simulink model "Send_IMU_value_I2C"  (R2016b)
settings: Solver=FixedStepAuto  StartTime=0.0  StopTime=10.0  RelTol=1e-3
PreLoadFcn:
  | waijung.modelPreload; % Required for working with Waijung Blockset. Do not remove.
undefined symbols (not defined in the file): deg_, g, imu, Link, LQFP100, ST, STM32F407VG, STM32F4DISCOVERY
libraries: simulink x20, stm32f4_i2c_lib x8, stm32f4_io_lib x3, BC_USB x2, stm32f4_device_config_lib x1
(part 1 of 2)
CloseFcn:
  | waijung.modelClose; % Required for working with Waijung Blockset. Do not remove.
settings Model: Creator=Wall  LastModifiedBy=Wall
settings OptimizationCC: DefaultParameterBehavior=Inlined
settings DebuggingCC: ParameterTunabilityLossMsg=error
settings HardwareCC: ProdBitPerPointer=32  ProdBitPerSizeT=32  ProdBitPerPtrDiffT=32  ProdLargestAtomicFloat=None  ProdIntDivRoundTo=Undefined  ProdWordSize=32  ProdHWDeviceType=ARM Compatible->Cortex - M4  TargetEndianess=LittleEndian  TargetHWDeviceType=ARM Compatible->Cortex - M4
settings RTWCC: SystemTargetFile=stm32f4.tlc  GenerateMakefile=off  TemplateMakefile=ert_default_tmf  Description=STM32F4 Target
settings CodeAppCC: ForceParamTrailComments=on  IgnoreCustomStorageClasses=off  OperatorAnnotations=on  SimulinkDataObjDesc=on  SFDataObjDesc=on  MATLABFcnDesc=on  InsertBlockDesc=on  MATLABSourceComments=on
settings STFCustomTargetCC: TargetLangStandard=C99 (ISO)  ModelReferenceCompliant=off  CombineOutputUpdateFcns=on  ERTCustomFileBanners=on  SupportContinuousTime=off  SupportNonInlinedSFcns=off  RemoveResetFunc=on  MATLABClassNameForMDSCustomization=Simulink.SoftwareTarget.ERTCustomization  GRTInterface=off  SystemTargetFile=stm32f4.tlc
settings ERTTargetCC: TargetLangStandard=C99 (ISO)  ModelReferenceCompliant=off  ParMdlRefBuildCompliant=off  CompOptLevelCompliant=off  ConcurrentExecutionCompliant=off  ERTFirstTimeCompliant=off  ModelStepFunctionPrototypeControlCompliant=off  CPPClassGenCompliant=off  UseToolchainInfoCompliant=off  InlinedParameterPlacement=NonHierarchical  ERTSrcFileBannerTemplate=stm32f4_code_template.cgt  ERTHdrFileBannerTemplate=stm32f4_code_template.cgt  ERTDataSrcFileTemplate=stm32f4_code_template.cgt  ERTDataHdrFileTemplate=stm32f4_code_template.cgt  ERTCustomFileTemplate=stm32f4_file_process.tlc

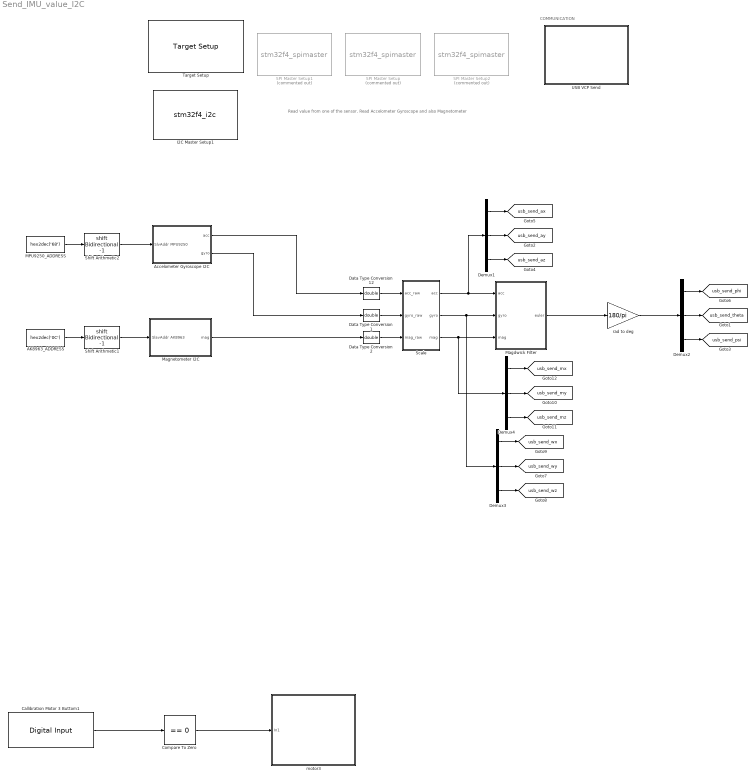
== system Send_IMU_value_I2C ==
  note: Read value from one of the sensor. Read Accelometer Gyroscope and also Magnetometer
  note: COMMUNICATION
  " AK8963_ADDRESS" : Constant  Value=hex2dec('0C')  OutDataTypeStr=uint8  SampleTime=0.002
  " MPU9250_ADDRESS" : Constant  Value=hex2dec('68')  OutDataTypeStr=uint8  SampleTime=0.002
  Accelometer Gyroscope I2C : Subsystem
  Callibration Motor 3 Buttom1 : stm32f4_io_lib/Digital Input  port=E  speed=100  porttype=Pull Up  porttypestr=UP  use_pin0=off  use_pin1=off  use_pin2=off  use_pin3=off  use_pin4=off  use_pin5=off  use_pin6=off  use_pin7=off  use_pin8=off  use_pin9=off  use_pin10=on  use_pin11=off  use_pin12=off  use_pin13=off  use_pin14=off  use_pin15=off  pinstr=GPIO_Pin_10  usedpinarray="[0  0  0  0  0  0  0  0  0  0  1  0  0  0  0  0]"  bitbandingstr="#define CallibrationMotor3Buttom1_E10 Peripheral_BB(GPIOE->IDR, 10)  /* Output pin */"  sampletime=0.002  sampletimestr=-1  blockid=CallibrationMotor3Buttom1  enablecustomportlabel=off  glabalinit=off  cinputportlabel=In1, In2  coutputportlabel=Out1, Out2
  Compare To Zero : simulink/Logic and Bit Operations/Compare To Zero  relop===  OutDataTypeStr=boolean
  Data Type Conversion1 : DataTypeConversion  OutDataTypeStr=double
  Data Type Conversion12 : DataTypeConversion  OutDataTypeStr=double
  Data Type Conversion2 : DataTypeConversion  OutDataTypeStr=double
  Demux{1..4} (4 alike) : Demux  Outputs=3
  I2C Master Setup1 : S-Function  FunctionName=stm32f4_i2c  Parameters=configuration,module,transfer,clkspeed,timeout,sdapin,sclpin,writecount,readcount,inputtypearray,outputtypearray,confstr,sampletime,sampletimestr,blockid  SFunctionDeploymentMode=off  EnableBusSupport=off  mask(stm32f4_i2c){configuration=Setup, module=1, lastmodule=1, transfer=Blocking, dutycycle=TLow/THigh = 2, clkspeed=400, timeout=25, writecount=0, readcount=0, sdapin=B9, sclpin=B6, waitwritetime=0, inputtypearray=[0], outputtypearray=[0], confstr=["B","9","B","6","1","1","6","0","I2C_DutyCycle_2","0","off"], sampletime=-1, sampletimestr=-1, blockid=I2CMasterSetup1}
      mask prompts: module "I2C Module"; lastmodule "Last module"; transfer "Transfer mode"; dutycycle "Duty cycle in fast mode"; clkspeed "Clock speed (kHz)"; timeout "Timeout (ms)"; writecount "Bytes write count"; readcount "Bytes read count"; sdapin "SDA pin"; sclpin "SCL pin"; waitwritetime "Wait write time (ms), default is 0"; inputtypearray "Input type array"; outputtypearray "Output type array"; confstr "Configuration string"; sampletime "Sample time (sec)"; sampletimestr "Compiled sample time (sec) in string"
      mask init:
      | stm32f4_i2c_callback('init');
      mask Help: web(fullfile(waijungdocroot,'stm32f4_i2c_setup.htm'), '-browser')
      mask TypeOptions configuration: Setup | Transaction
      mask Callback configuration: stm32f4_i2c_callback('configuration');
      mask TypeOptions module: 1 | 2 | 3
      mask Callback module: stm32f4_i2c_callback('module');
      mask TypeOptions transfer: Blocking | Non-blocking
      mask TypeOptions dutycycle: TLow/THigh = 16/9 | TLow/THigh = 2
      mask Callback dutycycle: stm32f4_i2c_callback('dutycycle');
      mask Callback writecount: stm32f4_i2c_callback('writecount');
      mask Callback readcount: stm32f4_i2c_callback('readcount');
      mask TypeOptions sdapin: - | B7 | B9
      mask Callback sdapin: stm32f4_i2c_callback('sdapin');
      mask TypeOptions sclpin: - | B6 | B8
      mask Callback sclpin: stm32f4_i2c_callback('sclpin');
      mask Callback confstr: stm32f4_i2c_callback('confstr');
      mask Callback sampletime: stm32f4_i2c_callback('sampletime');
      mask Callback sampletimestr: stm32f4_i2c_callback('sampletimestr');
      mask Callback blockid: stm32f4_i2c_callback('blockid');
      mask Display: text(0.5, 0.5, 'Module: I2C1\nClock: 400kHz\nSDA/SCL Pin: B9/B6','ver','middle','hor','center');
  Magdwick Filter : MATLAB Function  TreatAsAtomicUnit=on
  Magnetometer I2C : Subsystem
  SPI Master Setup : S-Function  Commented=on  FunctionName=stm32f4_spimaster  Parameters=mode,configuration,module,datacount,inputtypearray,outputtypearray,confstr,sampletime,sampletimestr,blockid  SFunctionDeploymentMode=off  EnableBusSupport=off  mask(stm32f4_spimaster){configuration=Setup, module=2, mode=Write, lastmodule=2, direction=Full-Duplex, dataformat=8bit/ FirstBit_MSB, prescaler=32, lastpclk=42000000, baudrate=1312500, cpolcpha=CPOL_Low/ CPHA_1Edge, datacount=0, nssmode=Software, nsspin=Not used, softnssport=B, softnsspin=12, sckpin=B13, misopin=B14, mosipin=B15, pintype=Push Pull, pulltype=Pull Up, nssdelay=0, inputtypearray=[0], outputtypearray=[0], confstr=["SPI_Direction_2Lines_FullDuplex","8b","MSB","Low","1Edge","32","Soft","0","x","x","1","B","12","1","B","13","1","B","14","1","B","15","0","1","0","0","0","0","0","0","0","PP","0","UP"], sampletime=-1, sampletimestr=0.002, blockid=SPIMasterSetup}
      mask prompts: module "SPI Module:"; lastmodule "Last module:"; dataformat "Data format:"; prescaler "Buad rate prescaler: Pclk/"; lastpclk "Last PCLK"; baudrate "Baud rate (Hz)"; cpolcpha "Clock polarity (CPOL)/ Clock phase (CPHA):"; datacount "Data Write count:"; nssmode "Slave/chip select (nSS, nCS) mode"; nsspin "Slave/chip select (nSS, nCS) pin"; softnssport "Slave/chip select port (nSS, nCS)"; softnsspin "Slave/chip select pin (nSS, nCS)"; sckpin "SCLK pin:"; misopin "MISO pin:"; mosipin "MOSI pin:"; pintype "Pin type (Push-Pull/Open-Drain)"; pulltype "Pull Type (Up/Down)"; nssdelay "Data delay time, uS:"; inputtypearray "Input type array"; outputtypearray "Output type array"; confstr "Configuration string"; sampletime "Sample time (sec)"; sampletimestr "Compiled sample time (sec) in string"
      mask help:
      | Direction:
      |  - Full-Duplex, use this mode when need to send and receive data at same clock.
      |  - Half-Duplex_Tx, this mode is to transmit data to slave only. Pin MISO (Rx) can be free for other function.
      |  - Half-Duplex_Rx, this mode is to receive data from slave only. Pin MOSIO (Tx) can be free for other function.
      | Data format:
      |   This configuration is depending on the specification of slave device.
      | Baud rate prescaler:
      |  - Use this prescaler to devide from the PCLK for SPI clock.
      |  - This Prescaler value is auto determine corresponding to baudrate setting and selected SPI module.
      | Baud rate (Hz):
      |  - Select baud rate for SPI clock. Please check the maximum clock support for target slave device.
      | Clock polarity and Clock phase:
      |  - This configuration parameter is depending on slave device.
      |  - See waijung help for more description.
      | Slave/chip select mode:
      |  - Hardware, use hardware SPI module for slave select (or chip select) pin.
      |  - Software, this mode allow any available pin for slave select (or chip select) function.
      |  - Custom, SPI block did not control slave select pin. User may use Digital Output block to control by costom.
      mask init:
      | stm32f4_spimaster_callback('init');
      mask Help: web(fullfile(waijungdocroot,'stm32f4_spimaster_setup.htm'), '-browser')
      mask TypeOptions configuration: Setup | Transaction
      mask Callback configuration: stm32f4_spimaster_callback('configuration');
      mask TypeOptions module: 1 | 2 | 3
      mask Callback module: stm32f4_spimaster_callback('module');
      mask TypeOptions mode: Read/ Write | Read | Write
      mask Callback mode: stm32f4_spimaster_callback('mode');
      mask TypeOptions direction: Full-Duplex | Half-Duplex_Tx | Half-Duplex_Rx
      mask Callback direction: stm32f4_spimaster_callback('direction');
      mask TypeOptions dataformat: 8bit/ FirstBit_MSB | 8bit/ FirstBit_LSB | 16bit/ FirstBit_MSB | 16bit/ FirstBit_LSB
      mask TypeOptions prescaler: 2 | 4 | 8 | 16 | 32 | 64 | 128 | 256
      mask TypeOptions baudrate: Not set | 21000000 | 10500000 | 5250000 | 2625000 | 1312500 | 656250 | 328125 | 164063
      mask Callback baudrate: stm32f4_spimaster_callback('baudrate');
      mask TypeOptions cpolcpha: CPOL_Low/ CPHA_1Edge | CPOL_Low/ CPHA_2Edge | CPOL_High/ CPHA_1Edge | CPOL_High/ CPHA_2Edge
      mask Callback datacount: stm32f4_spimaster_callback('datacount');
      mask TypeOptions nssmode: Hardware | Software | Custom
      mask Callback nssmode: stm32f4_spimaster_callback('nssmode');
      mask TypeOptions nsspin: Not used | B9 | B12
      mask TypeOptions softnssport: A | B | C | D | E | F | G | H | I
      mask TypeOptions softnsspin: 0 | 1 | 2 | 3 | 4 | 5 | 6 | 7 | 8 | 9 | 10 | 11 | 12 | 13 | 14 | 15
      mask TypeOptions sckpin: Not used | B10 | B13
      mask TypeOptions misopin: Not used | B14 | C2
      mask TypeOptions mosipin: Not used | B15 | C3
      mask TypeOptions pintype: Push Pull | Open Drain
      mask TypeOptions pulltype: None | Pull Up | Pull Down
      mask Callback confstr: stm32f4_spimaster_callback('confstr');
      mask Callback sampletime: stm32f4_spimaster_callback('sampletime');
      mask Callback sampletimestr: stm32f4_spimaster_callback('sampletimestr');
      mask Callback blockid: stm32f4_spimaster_callback('blockid');
      mask Display: text(0.5, 0.5, 'Module: SPI2 (Master)\nFull-Duplex\nBaudrate: 1312500','ver','middle','hor','center');
  SPI Master Setup1 : S-Function  Commented=on  FunctionName=stm32f4_spimaster  Parameters=mode,configuration,module,datacount,inputtypearray,outputtypearray,confstr,sampletime,sampletimestr,blockid  SFunctionDeploymentMode=off  EnableBusSupport=off  mask(stm32f4_spimaster){configuration=Setup, module=1, mode=Write, lastmodule=1, direction=Full-Duplex, dataformat=8bit/ FirstBit_MSB, prescaler=64, lastpclk=84000000, baudrate=1312500, cpolcpha=CPOL_Low/ CPHA_1Edge, datacount=0, nssmode=Software, nsspin=Not used, softnssport=C, softnsspin=5, sckpin=A5, misopin=A6, mosipin=A7, pintype=Push Pull, pulltype=Pull Up, nssdelay=0, inputtypearray=[0], outputtypearray=[0], confstr=["SPI_Direction_2Lines_FullDuplex","8b","MSB","Low","1Edge","64","Soft","0","x","x","1","C","5","1","A","5","1","A","6","1","A","7","1","0","1","0","0","0","0","0","0","PP","0","UP"], sampletime=-1, sampletimestr=0.002, blockid=SPIMasterSetup1}
      mask prompts: module "SPI Module:"; lastmodule "Last module:"; dataformat "Data format:"; prescaler "Buad rate prescaler: Pclk/"; lastpclk "Last PCLK"; baudrate "Baud rate (Hz)"; cpolcpha "Clock polarity (CPOL)/ Clock phase (CPHA):"; datacount "Data Write count:"; nssmode "Slave/chip select (nSS, nCS) mode"; nsspin "Slave/chip select (nSS, nCS) pin"; softnssport "Slave/chip select port (nSS, nCS)"; softnsspin "Slave/chip select pin (nSS, nCS)"; sckpin "SCLK pin:"; misopin "MISO pin:"; mosipin "MOSI pin:"; pintype "Pin type (Push-Pull/Open-Drain)"; pulltype "Pull Type (Up/Down)"; nssdelay "Data delay time, uS:"; inputtypearray "Input type array"; outputtypearray "Output type array"; confstr "Configuration string"; sampletime "Sample time (sec)"; sampletimestr "Compiled sample time (sec) in string"
      mask help:
      | Direction:
      |  - Full-Duplex, use this mode when need to send and receive data at same clock.
      |  - Half-Duplex_Tx, this mode is to transmit data to slave only. Pin MISO (Rx) can be free for other function.
      |  - Half-Duplex_Rx, this mode is to receive data from slave only. Pin MOSIO (Tx) can be free for other function.
      | Data format:
      |   This configuration is depending on the specification of slave device.
      | Baud rate prescaler:
      |  - Use this prescaler to devide from the PCLK for SPI clock.
      |  - This Prescaler value is auto determine corresponding to baudrate setting and selected SPI module.
      | Baud rate (Hz):
      |  - Select baud rate for SPI clock. Please check the maximum clock support for target slave device.
      | Clock polarity and Clock phase:
      |  - This configuration parameter is depending on slave device.
      |  - See waijung help for more description.
      | Slave/chip select mode:
      |  - Hardware, use hardware SPI module for slave select (or chip select) pin.
      |  - Software, this mode allow any available pin for slave select (or chip select) function.
      |  - Custom, SPI block did not control slave select pin. User may use Digital Output block to control by costom.
      mask init:
      | stm32f4_spimaster_callback('init');
      mask Help: web(fullfile(waijungdocroot,'stm32f4_spimaster_setup.htm'), '-browser')
      mask TypeOptions configuration: Setup | Transaction
      mask Callback configuration: stm32f4_spimaster_callback('configuration');
      mask TypeOptions module: 1 | 2 | 3
      mask Callback module: stm32f4_spimaster_callback('module');
      mask TypeOptions mode: Read/ Write | Read | Write
      mask Callback mode: stm32f4_spimaster_callback('mode');
      mask TypeOptions direction: Full-Duplex | Half-Duplex_Tx | Half-Duplex_Rx
      mask Callback direction: stm32f4_spimaster_callback('direction');
      mask TypeOptions dataformat: 8bit/ FirstBit_MSB | 8bit/ FirstBit_LSB | 16bit/ FirstBit_MSB | 16bit/ FirstBit_LSB
      mask TypeOptions prescaler: 2 | 4 | 8 | 16 | 32 | 64 | 128 | 256
      mask TypeOptions baudrate: Not set | 42000000 | 21000000 | 10500000 | 5250000 | 2625000 | 1312500 | 656250 | 328125
      mask Callback baudrate: stm32f4_spimaster_callback('baudrate');
      mask TypeOptions cpolcpha: CPOL_Low/ CPHA_1Edge | CPOL_Low/ CPHA_2Edge | CPOL_High/ CPHA_1Edge | CPOL_High/ CPHA_2Edge
      mask Callback datacount: stm32f4_spimaster_callback('datacount');
      mask TypeOptions nssmode: Hardware | Software | Custom
      mask Callback nssmode: stm32f4_spimaster_callback('nssmode');
      mask TypeOptions nsspin: Not used | A4 | A15
      mask TypeOptions softnssport: A | B | C | D | E | F | G | H | I
      mask TypeOptions softnsspin: 0 | 1 | 2 | 3 | 4 | 5 | 6 | 7 | 8 | 9 | 10 | 11 | 12 | 13 | 14 | 15
      mask TypeOptions sckpin: Not used | A5 | B3
      mask TypeOptions misopin: Not used | A6 | B4
      mask TypeOptions mosipin: Not used | A7 | B5
      mask TypeOptions pintype: Push Pull | Open Drain
      mask TypeOptions pulltype: None | Pull Up | Pull Down
      mask Callback confstr: stm32f4_spimaster_callback('confstr');
      mask Callback sampletime: stm32f4_spimaster_callback('sampletime');
      mask Callback sampletimestr: stm32f4_spimaster_callback('sampletimestr');
      mask Callback blockid: stm32f4_spimaster_callback('blockid');
      mask Display: text(0.5, 0.5, 'Module: SPI1 (Master)\nFull-Duplex\nBaudrate: 1312500','ver','middle','hor','center');
  SPI Master Setup2 : S-Function  Commented=on  FunctionName=stm32f4_spimaster  Parameters=mode,configuration,module,datacount,inputtypearray,outputtypearray,confstr,sampletime,sampletimestr,blockid  SFunctionDeploymentMode=off  EnableBusSupport=off  mask(stm32f4_spimaster){configuration=Setup, module=3, mode=Write, lastmodule=3, direction=Full-Duplex, dataformat=8bit/ FirstBit_MSB, prescaler=32, lastpclk=42000000, baudrate=1312500, cpolcpha=CPOL_Low/ CPHA_1Edge, datacount=0, nssmode=Software, nsspin=Not used, softnssport=C, softnsspin=11, sckpin=C10, misopin=B4, mosipin=B5, pintype=Push Pull, pulltype=Pull Up, nssdelay=0, inputtypearray=[0], outputtypearray=[0], confstr=["SPI_Direction_2Lines_FullDuplex","8b","MSB","Low","1Edge","32","Soft","0","x","x","1","C","11","1","C","10","1","B","4","1","B","5","0","1","1","0","0","0","0","0","0","PP","0","UP"], sampletime=-1, sampletimestr=0.002, blockid=SPIMasterSetup2}
      mask prompts: module "SPI Module:"; lastmodule "Last module:"; dataformat "Data format:"; prescaler "Buad rate prescaler: Pclk/"; lastpclk "Last PCLK"; baudrate "Baud rate (Hz)"; cpolcpha "Clock polarity (CPOL)/ Clock phase (CPHA):"; datacount "Data Write count:"; nssmode "Slave/chip select (nSS, nCS) mode"; nsspin "Slave/chip select (nSS, nCS) pin"; softnssport "Slave/chip select port (nSS, nCS)"; softnsspin "Slave/chip select pin (nSS, nCS)"; sckpin "SCLK pin:"; misopin "MISO pin:"; mosipin "MOSI pin:"; pintype "Pin type (Push-Pull/Open-Drain)"; pulltype "Pull Type (Up/Down)"; nssdelay "Data delay time, uS:"; inputtypearray "Input type array"; outputtypearray "Output type array"; confstr "Configuration string"; sampletime "Sample time (sec)"; sampletimestr "Compiled sample time (sec) in string"
      mask help:
      | Direction:
      |  - Full-Duplex, use this mode when need to send and receive data at same clock.
      |  - Half-Duplex_Tx, this mode is to transmit data to slave only. Pin MISO (Rx) can be free for other function.
      |  - Half-Duplex_Rx, this mode is to receive data from slave only. Pin MOSIO (Tx) can be free for other function.
      | Data format:
      |   This configuration is depending on the specification of slave device.
      | Baud rate prescaler:
      |  - Use this prescaler to devide from the PCLK for SPI clock.
      |  - This Prescaler value is auto determine corresponding to baudrate setting and selected SPI module.
      | Baud rate (Hz):
      |  - Select baud rate for SPI clock. Please check the maximum clock support for target slave device.
      | Clock polarity and Clock phase:
      |  - This configuration parameter is depending on slave device.
      |  - See waijung help for more description.
      | Slave/chip select mode:
      |  - Hardware, use hardware SPI module for slave select (or chip select) pin.
      |  - Software, this mode allow any available pin for slave select (or chip select) function.
      |  - Custom, SPI block did not control slave select pin. User may use Digital Output block to control by costom.
      mask init:
      | stm32f4_spimaster_callback('init');
      mask Help: web(fullfile(waijungdocroot,'stm32f4_spimaster_setup.htm'), '-browser')
      mask TypeOptions configuration: Setup | Transaction
      mask Callback configuration: stm32f4_spimaster_callback('configuration');
      mask TypeOptions module: 1 | 2 | 3
      mask Callback module: stm32f4_spimaster_callback('module');
      mask TypeOptions mode: Read/ Write | Read | Write
      mask Callback mode: stm32f4_spimaster_callback('mode');
      mask TypeOptions direction: Full-Duplex | Half-Duplex_Tx | Half-Duplex_Rx
      mask Callback direction: stm32f4_spimaster_callback('direction');
      mask TypeOptions dataformat: 8bit/ FirstBit_MSB | 8bit/ FirstBit_LSB | 16bit/ FirstBit_MSB | 16bit/ FirstBit_LSB
      mask TypeOptions prescaler: 2 | 4 | 8 | 16 | 32 | 64 | 128 | 256
      mask TypeOptions baudrate: Not set | 21000000 | 10500000 | 5250000 | 2625000 | 1312500 | 656250 | 328125 | 164063
      mask Callback baudrate: stm32f4_spimaster_callback('baudrate');
      mask TypeOptions cpolcpha: CPOL_Low/ CPHA_1Edge | CPOL_Low/ CPHA_2Edge | CPOL_High/ CPHA_1Edge | CPOL_High/ CPHA_2Edge
      mask Callback datacount: stm32f4_spimaster_callback('datacount');
      mask TypeOptions nssmode: Hardware | Software | Custom
      mask Callback nssmode: stm32f4_spimaster_callback('nssmode');
      mask TypeOptions nsspin: Not used | A4 | A15
      mask TypeOptions softnssport: A | B | C | D | E | F | G | H | I
      mask TypeOptions softnsspin: 0 | 1 | 2 | 3 | 4 | 5 | 6 | 7 | 8 | 9 | 10 | 11 | 12 | 13 | 14 | 15
      mask TypeOptions sckpin: Not used | B3 | C10
      mask TypeOptions misopin: Not used | B4 | C11
      mask TypeOptions mosipin: Not used | B5 | C12
      mask TypeOptions pintype: Push Pull | Open Drain
      mask TypeOptions pulltype: None | Pull Up | Pull Down
      mask Callback confstr: stm32f4_spimaster_callback('confstr');
      mask Callback sampletime: stm32f4_spimaster_callback('sampletime');
      mask Callback sampletimestr: stm32f4_spimaster_callback('sampletimestr');
      mask Callback blockid: stm32f4_spimaster_callback('blockid');
      mask Display: text(0.5, 0.5, 'Module: SPI3 (Master)\nFull-Duplex\nBaudrate: 1312500','ver','middle','hor','center');
  Scale : Subsystem
  Shift Arithmetic1 : ArithShift  BitShiftNumber=-1
  Shift Arithmetic2 : ArithShift  BitShiftNumber=-1
  Target Setup : stm32f4_device_config_lib/Target Setup  Priority=100  compiler=GNU ARM  previous_compiler=GNU ARM  mcu=STM32F407VG (LQFP100); STM32F4DISCOVERY  mcustr=STM32F407VG  clockconfig=STM32F4DISCOVERY Default (HSEOSC-8MHz/HCLK-168MHz)  system_stm32f4xx_c_path=C:\waijung15_04a\targets\stm32f4_target\stm32f4\utils\STM32F4xx_AN3988_V1.0.1\stm32f4_default\hseosc8mhz  showmemoryconfiguration=off  stacksize=0x400  heapsize=0x200  enableautocompiledownload=on  fullchiperase=off  programmerinterface=ST-Link  editctrlstr=on  compilercontrolstr=$(patsubst %, -I%, .) -mcpu=cortex-m4 -mthumb -mthumb-interwork -mfloat-abi=hard -mfpu=fpv4-sp-d16 -ffast-math -Wall -Wextra -Ofast  assemblercontrolstr=$(patsubst %, -I%, .) -mcpu=cortex-m4 -mthumb -mthumb-interwork -mfloat-abi=hard -mfpu=fpv4-sp-d16 -ffast-math -Wall -Wextra -Ofast -Wa,-amhls=$(<:.s=.lst) -D__STACK_SIZE=$(STACK_SIZE) -D__HEAP_SIZE=$(HEAP_SIZE)  linkercontrolstr=-T$(LD_SCRIPT) -g -Wl,-Map=$(MAP),--cref,--no-warn-mismatch -mcpu=cortex-m4 -mthumb -mthumb-interwork -mfloat-abi=hard -mfpu=fpv4-sp-d16  runafterdownload=on  execprofile=None  profileruart=1  profilerbaud=115200  profilertxpin=Not used  profilerinitstr=0.002,168000000,336000,115200,0  manualsetsampletime=on  sampletime=0.002  blockid=TargetSetup  systickreloadvalue=336000  hseval=8000000  lastprofileruart=1  hclk=168000000  flashorigin=0x8000000  flashlength=1M  ramorigin=0x20000000  ramlength=112k  useextram=off
  USB VCP Send : Subsystem
  motor3 : Subsystem
  rad to deg : Gain  Gain=180/pi
  tag scope: usb_send_ax=global, usb_send_ay=global, usb_send_az=global, usb_send_mx=global, usb_send_my=global, usb_send_mz=global, usb_send_phi=global, usb_send_psi=global, usb_send_theta=global, usb_send_wx=global, usb_send_wy=global, usb_send_wz=global
  wires:
  Demux2/1 -> [usb_send_phi]
  Demux2/2 -> [usb_send_theta]
  Demux2/3 -> [usb_send_psi]
  Demux1/1 -> [usb_send_ax]
  Demux1/2 -> [usb_send_ay]
  Demux1/3 -> [usb_send_az]
  Demux3/1 -> [usb_send_wx]
  Demux3/2 -> [usb_send_wy]
  Demux3/3 -> [usb_send_wz]
  Scale/2(gyro) -> Demux3/1, Magdwick Filter/2(gyro)
  Scale/1(acc) -> Demux1/1, Magdwick Filter/1(acc)
  Demux4/1 -> [usb_send_mx]
  Demux4/2 -> [usb_send_my]
  Demux4/3 -> [usb_send_mz]
  Data Type Conversion12/1 -> Scale/1(acc_raw)
  Data Type Conversion1/1 -> Scale/2(gyro_raw)
  " MPU9250_ADDRESS"/1 -> Shift Arithmetic2/1
  " AK8963_ADDRESS"/1 -> Shift Arithmetic1/1
  Shift Arithmetic1/1 -> Magnetometer I2C/1(SlavAddr AK8963)
  Shift Arithmetic2/1 -> Accelometer Gyroscope I2C/1(SlvAddr MPU9250)
  Data Type Conversion2/1 -> Scale/3(mag_raw)
  Scale/3(mag) -> Demux4/1, Magdwick Filter/3(mag)
  Magnetometer I2C/1(mag) -> Data Type Conversion2/1
  Accelometer Gyroscope I2C/2(gyro) -> Data Type Conversion1/1
  Accelometer Gyroscope I2C/1(acc) -> Data Type Conversion12/1
  Callibration Motor 3 Buttom1/1 -> Compare To Zero/1
  Compare To Zero/1 -> motor3/1(In1)
  Magdwick Filter/1(euler) -> rad to deg/1
  rad to deg/1 -> Demux2/1

== system Send_IMU_value_I2C/Accelometer Gyroscope I2C ==
  SlvAddr MPU9250 : Inport
  MPU9250 Init : Subsystem
  Read Accelometer and Gyroscope Data : Subsystem
  acc : Outport
  gyro : Outport  Port=2
  wires:
  SlvAddr MPU9250/1 -> Read Accelometer and Gyroscope Data/1(SlvAddr), MPU9250 Init/1(SlvAddr)
  Read Accelometer and Gyroscope Data/1(acc) -> acc/1
  Read Accelometer and Gyroscope Data/2(gyro) -> gyro/1
  MPU9250 Init/1(SETUP_READY) -> Read Accelometer and Gyroscope Data/Enable

== system Send_IMU_value_I2C/Magnetometer I2C ==
  SlavAddr AK8963 : Inport
  "AK8963 Init " : Subsystem
  "Magnetometer Data Ready " : Subsystem
  Read Magnetometer Data : Subsystem
  mag : Outport
  wires:
  "AK8963 Init "/1(READY) -> "Magnetometer Data Ready "/Enable
  Read Magnetometer Data/1(mag) -> mag/1
  SlavAddr AK8963/1 -> "Magnetometer Data Ready "/1(SlvAddr), Read Magnetometer Data/1("SlvAddr "), "AK8963 Init "/1(SlvAddr)
  "Magnetometer Data Ready "/1(READY) -> Read Magnetometer Data/Enable

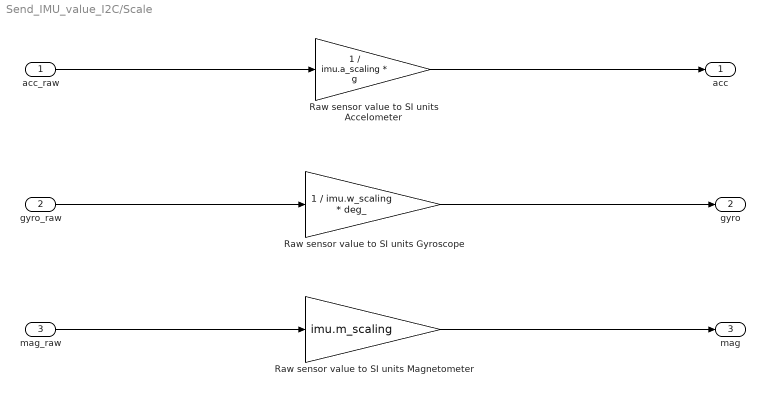
== system Send_IMU_value_I2C/Scale ==
  acc_raw : Inport
  gyro_raw : Inport  Port=2
  mag_raw : Inport  Port=3
  Raw sensor value to SI units Accelometer : Gain  Gain=1 / imu.a_scaling * g
  Raw sensor value to SI units Gyroscope : Gain  Gain=1 / imu.w_scaling * deg_
  Raw sensor value to SI units Magnetometer : Gain  Gain=imu.m_scaling
  acc : Outport
  gyro : Outport  Port=2
  mag : Outport  Port=3
  wires:
  gyro_raw/1 -> Raw sensor value to SI units Gyroscope/1
  Raw sensor value to SI units Accelometer/1 -> acc/1
  Raw sensor value to SI units Gyroscope/1 -> gyro/1
  acc_raw/1 -> Raw sensor value to SI units Accelometer/1
  mag_raw/1 -> Raw sensor value to SI units Magnetometer/1
  Raw sensor value to SI units Magnetometer/1 -> mag/1

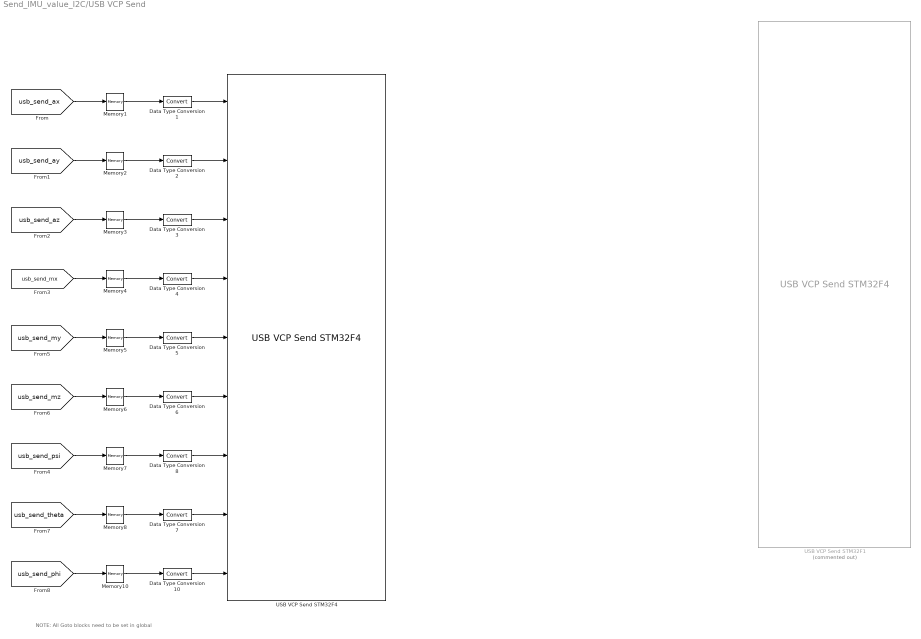
== system Send_IMU_value_I2C/USB VCP Send ==
  note: NOTE: All Goto blocks need to be set in global
  Data Type Conversion{1..8,10} (9 alike) : DataTypeConversion
  Memory{1..8,10} (9 alike) : Memory  InheritSampleTime=on
  USB VCP Send STM32F1 : BC_USB/USB VCP Send STM32F4  Commented=on  speed="USB 1.1   12Mbit/s"  data_size=2048 Bytes  header_data='0E 0E'  binary_data='double double double double double double double double double'  terminator_data='0A 0A'  sampletime=Ts
  USB VCP Send STM32F4 : BC_USB/USB VCP Send STM32F4  speed="USB 1.1   12Mbit/s"  data_size=2048 Bytes  header_data='0E 0E'  binary_data='double double double double double double double double double'  terminator_data='0A 0A'  sampletime=0.002
  wires:
  Memory7/1 -> Data Type Conversion8/1
  Data Type Conversion8/1 -> USB VCP Send STM32F4/7
  Data Type Conversion1/1 -> USB VCP Send STM32F4/1
  Memory2/1 -> Data Type Conversion2/1
  Memory1/1 -> Data Type Conversion1/1
  [usb_send_ax] -> Memory1/1
  Data Type Conversion2/1 -> USB VCP Send STM32F4/2
  Memory6/1 -> Data Type Conversion6/1
  Data Type Conversion3/1 -> USB VCP Send STM32F4/3
  [usb_send_ay] -> Memory2/1
  [usb_send_az] -> Memory3/1
  Memory3/1 -> Data Type Conversion3/1
  Memory4/1 -> Data Type Conversion4/1
  [usb_send_mx] -> Memory4/1
  Data Type Conversion4/1 -> USB VCP Send STM32F4/4
  Memory5/1 -> Data Type Conversion5/1
  Data Type Conversion5/1 -> USB VCP Send STM32F4/5
  Data Type Conversion6/1 -> USB VCP Send STM32F4/6
  [usb_send_my] -> Memory5/1
  [usb_send_psi] -> Memory7/1
  [usb_send_mz] -> Memory6/1
  Memory8/1 -> Data Type Conversion7/1
  Data Type Conversion7/1 -> USB VCP Send STM32F4/8
  [usb_send_theta] -> Memory8/1
  Memory10/1 -> Data Type Conversion10/1
  Data Type Conversion10/1 -> USB VCP Send STM32F4/9
  [usb_send_phi] -> Memory10/1

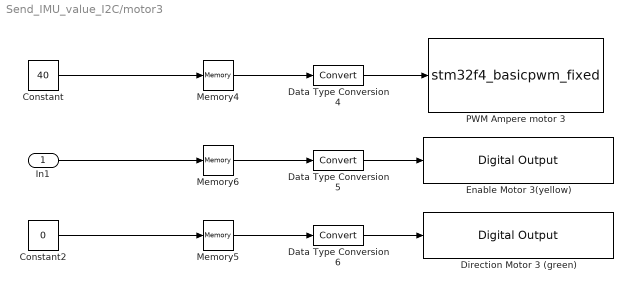
== system Send_IMU_value_I2C/motor3 ==
  In1 : Inport
  Constant : Constant  Value=40
  Constant2 : Constant  Value=0
  Data Type Conversion4 : DataTypeConversion
  Data Type Conversion5 : DataTypeConversion
  Data Type Conversion6 : DataTypeConversion
  Direction Motor 3 (green) : stm32f4_io_lib/Digital Output  use_bitband=on  port=D  speed=100  porttype=Push Pull  porttypestr=PP  use_pin0=off  use_pin1=off  use_pin2=off  use_pin3=off  use_pin4=off  use_pin5=off  use_pin6=off  use_pin7=off  use_pin8=off  use_pin9=off  use_pin10=off  use_pin11=on  use_pin12=off  use_pin13=off  use_pin14=off  use_pin15=off  pinstr=GPIO_Pin_11  usedpinarray="[0  0  0  0  0  0  0  0  0  0  0  1  0  0  0  0]"  bitbandingstr="#define motor3DirectionMotor3green_D11 Peripheral_BB(GPIOD->ODR, 11)  /* Output pin */"  sampletime=-1  sampletimestr=-1  blockid=motor3DirectionMotor3green  enablecustomportlabel=off  globalinit=off  cinputportlabel=In1, In2  coutputportlabel=0
  Enable Motor 3(yellow) : stm32f4_io_lib/Digital Output  use_bitband=on  port=D  speed=100  porttype=Push Pull  porttypestr=PP  use_pin0=off  use_pin1=off  use_pin2=off  use_pin3=off  use_pin4=off  use_pin5=off  use_pin6=off  use_pin7=off  use_pin8=off  use_pin9=on  use_pin10=off  use_pin11=off  use_pin12=off  use_pin13=off  use_pin14=off  use_pin15=off  pinstr=GPIO_Pin_9  usedpinarray="[0  0  0  0  0  0  0  0  0  1  0  0  0  0  0  0]"  bitbandingstr="#define motor3EnableMotor3yellow_D9 Peripheral_BB(GPIOD->ODR, 9)  /* Output pin */"  sampletime=-1  sampletimestr=-1  blockid=motor3EnableMotor3yellow  enablecustomportlabel=off  globalinit=off  cinputportlabel=In1, In2  coutputportlabel=0
  Memory4 : Memory  InheritSampleTime=on
  Memory5 : Memory  InheritSampleTime=on
  Memory6 : Memory  InheritSampleTime=on
  PWM Ampere motor 3 : S-Function  FunctionName=stm32f4_basicpwm_fixed  Parameters=timer,pwmperiod,uc3m_pwmperiod,ch1pin,ch2pin,ch3pin,ch4pin,sampletime,sampletimestr,blockid,apb,portstr,pinstr,pinmat,timarr,timprescale,chmat,polaritystr  SFunctionDeploymentMode=off  EnableBusSupport=off  mask(stm32f4_basicpwm_fixed){timer=2, pwmperiod=0.02, uc3m_pwmperiod=0.0002, polarity=Active High, polaritystr=TIM_OCPolarity_High, ch1pin=Not available - Do not use, ch2pin=Not available - Do not use, ch3pin=Not available - Do not use, ch4pin=A3, sampletime=0.002, sampletimestr=-1, blockid=motor3PWMAmperemotor3, portpinstr=,,,A3, enablecustomportlabel=off, cinputportlabel=In1, In2, In3, In4, coutputportlabel=0, callbackgensrccode=off, apb=1, portstr=["A"], pinstr=["GPIO_Pin_3"], pinmat=[1 3], timarr=59999, timprescale=55, chmat=[4]}
      mask prompts: pwmperiod "PWM Period (seconds)"; uc3m_pwmperiod "PWM Signal Period (seconds)"; ch1pin "Channel 1"; ch2pin "Channel 2"; ch3pin "Channel 3"; ch4pin "Channel 4"; sampletime "Sample time (sec)"; sampletimestr "Compiled sample time (sec) in string"; portpinstr "Port pin string"; enablecustomportlabel "Enable custom port labels"; cinputportlabel "Custom input port labels (Ex. In1, In2, In3)"; coutputportlabel "Custom output port labels (Ex. Out1, Out2, Out3)"; callbackgensrccode "Gen source code from callback"; portstr "Port string"; pinstr "Pin string"; pinmat "Pin matrix"; timarr "Timer ARR"; timprescale "Timer PRESCALE"; chmat "Channel order"
      mask help:
      | This block implements basic Edge-aligned Pulse Width Modulation (PWM) generation.
      | All timers are 16-bit. The PWM period is fixed (per timer).
      |
      | This block was fixed by Sr Antonio
      mask init:
      | stm32f4_basicpwm_callback_fixed('init');
      mask Help: web(fullfile(waijungdocroot,'stm32f4_basicpwm.htm'),'-browser')
      mask TypeOptions timer: 1 | 2 | 3 | 4 | 5 | 8 | 9 | 10 | 11 | 12 | 13 | 14
      mask Callback timer: stm32f4_basicpwm_callback_fixed('timer');
      mask Callback pwmperiod: stm32f4_basicpwm_callback_fixed('pwmperiod');
      mask Callback uc3m_pwmperiod: stm32f4_basicpwm_callback_fixed('uc3m_pwmperiod');
      mask TypeOptions polarity: Active High | Active Low
      mask Callback polarity: stm32f4_basicpwm_callback_fixed('polarity');
      mask TypeOptions ch1pin: Not available - Do not use | A0 | A5
      mask Callback ch1pin: stm32f4_basicpwm_callback_fixed('ch1pin');
      mask TypeOptions ch2pin: Not available - Do not use | A1 | B3
      mask Callback ch2pin: stm32f4_basicpwm_callback_fixed('ch2pin');
      mask TypeOptions ch3pin: Not available - Do not use | A2 | B10
      mask Callback ch3pin: stm32f4_basicpwm_callback_fixed('ch3pin');
      mask TypeOptions ch4pin: Not available - Do not use | A3 | B11
      mask Callback ch4pin: stm32f4_basicpwm_callback_fixed('ch4pin');
      mask Callback sampletime: stm32f4_basicpwm_callback_fixed('sampletime');
      mask Callback sampletimestr: stm32f4_basicpwm_callback_fixed('sampletimestr');
      mask Callback blockid: stm32f4_basicpwm_callback_fixed('blockid');
      mask Callback enablecustomportlabel: stm32f4_basicpwm_callback_fixed('enablecustomportlabel')
      mask Display: text(0.95, 0.5, 'UC3M FIXED\nTimer: 2\nPolarity: Active High\nPeriod (sec): 0.0002\nTs (sec): 0.002','ver','middle','hor','right');port_label('input', 1,'CH4 (A3)')
  wires:
  Constant/1 -> Memory4/1
  Data Type Conversion6/1 -> Direction Motor 3 (green)/1
  Data Type Conversion5/1 -> Enable Motor 3(yellow)/1
  Memory4/1 -> Data Type Conversion4/1
  Memory6/1 -> Data Type Conversion5/1
  Constant2/1 -> Memory5/1
  Memory5/1 -> Data Type Conversion6/1
  In1/1 -> Memory6/1
  Data Type Conversion4/1 -> PWM Ampere motor 3/1

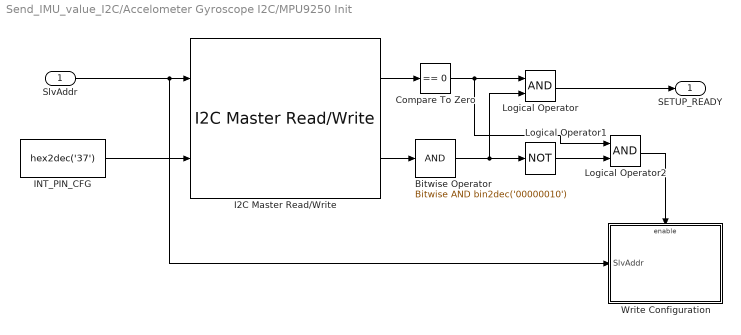
== system Send_IMU_value_I2C/Accelometer Gyroscope I2C/MPU9250 Init ==
  SlvAddr : Inport
  Bitwise Operator : simulink/Logic and Bit Operations/Bitwise Operator  logicop=AND  UseBitMask=on  BitMask=bin2dec('00000010')  BitMaskRealWorld=Stored Integer
  Compare To Zero : simulink/Logic and Bit Operations/Compare To Zero  relop===  OutDataTypeStr=boolean
  I2C Master Read/Write : stm32f4_i2c_lib/I2C Master Read//Write  configuration=Transaction  module=1  lastmodule=3  transfer=Blocking  dutycycle=TLow/THigh = 2  clkspeed=400  timeout=25  writecount=1  readcount=1  sdapin=C9  sclpin=A8  waitwritetime=0  forcestop=off  inputtypearray=[2 3 3]  outputtypearray=[2 3 3]  confstr="[\"C\",\"9\",\"A\",\"8\",\"1\",\"1\",\"6\",\"0\",\"I2C_DutyCycle_2\",\"0\",\"off\"]"  sampletime=-1  sampletimestr=-1  blockid=AccelometerGyroscopeI2CMPU9250InitI2CMasterReadWrite
  INT_PIN_CFG : Constant  Value=hex2dec('37')  OutDataTypeStr=uint8  SampleTime=-1
  Logical Operator : Logic  AllPortsSameDT=off  OutDataTypeStr=boolean
  Logical Operator1 : Logic  Operator=NOT  AllPortsSameDT=off  OutDataTypeStr=boolean
  Logical Operator2 : Logic  AllPortsSameDT=off  OutDataTypeStr=boolean
  Write Configuration : Subsystem
  SETUP_READY : Outport
  wires:
  I2C Master Read/Write/1 -> Compare To Zero/1
  INT_PIN_CFG/1 -> I2C Master Read/Write/2
  SlvAddr/1 -> Write Configuration/1(SlvAddr), I2C Master Read/Write/1
  Logical Operator/1 -> SETUP_READY/1
  Compare To Zero/1 -> Logical Operator2/1, Logical Operator/1
  Bitwise Operator/1 -> Logical Operator1/1, Logical Operator/2
  Logical Operator1/1 -> Logical Operator2/2
  Logical Operator2/1 -> Write Configuration/Enable
  I2C Master Read/Write/2 -> Bitwise Operator/1

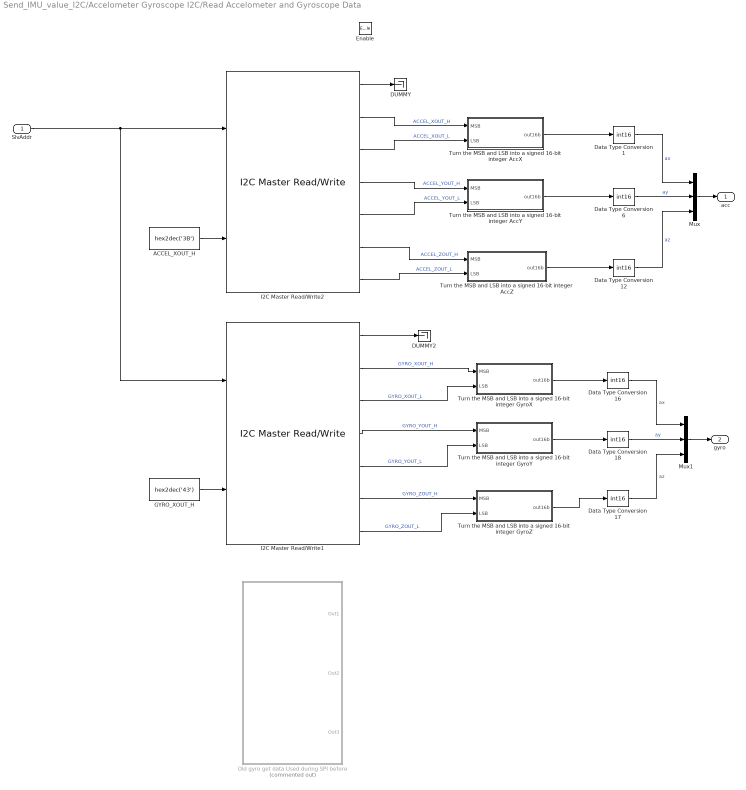
== system Send_IMU_value_I2C/Accelometer Gyroscope I2C/Read Accelometer and Gyroscope Data ==
  SlvAddr : Inport
  Enable : EnablePort
  ACCEL_XOUT_H : Constant  Value=hex2dec('3B')  OutDataTypeStr=uint8  SampleTime=-1
  DUMMY : Terminator
  DUMMY2 : Terminator
  Data Type Conversion{1,6,12,16..18} (6 alike) : DataTypeConversion  OutDataTypeStr=int16
  GYRO_XOUT_H : Constant  Value=hex2dec('43')  OutDataTypeStr=uint8  SampleTime=-1
  I2C Master Read/Write1 : stm32f4_i2c_lib/I2C Master Read//Write  configuration=Transaction  module=1  lastmodule=3  transfer=Blocking  dutycycle=TLow/THigh = 2  clkspeed=400  timeout=25  writecount=1  readcount=6  sdapin=C9  sclpin=A8  waitwritetime=0  forcestop=off  inputtypearray=[2 3 3]  outputtypearray=[7 3 3 3 3 3 3 3]  confstr="[\"C\",\"9\",\"A\",\"8\",\"1\",\"1\",\"6\",\"0\",\"I2C_DutyCycle_2\",\"0\",\"off\"]"  sampletime=-1  sampletimestr=-1  blockid=AccelometerGyroscopeI2CReadAccelometerandGyroscopeDataI2CMasterReadWrite1
  I2C Master Read/Write2 : stm32f4_i2c_lib/I2C Master Read//Write  configuration=Transaction  module=1  lastmodule=3  transfer=Blocking  dutycycle=TLow/THigh = 2  clkspeed=400  timeout=25  writecount=1  readcount=6  sdapin=C9  sclpin=A8  waitwritetime=0  forcestop=off  inputtypearray=[2 3 3]  outputtypearray=[7 3 3 3 3 3 3 3]  confstr="[\"C\",\"9\",\"A\",\"8\",\"1\",\"1\",\"6\",\"0\",\"I2C_DutyCycle_2\",\"0\",\"off\"]"  sampletime=-1  sampletimestr=-1  blockid=AccelometerGyroscopeI2CReadAccelometerandGyroscopeDataI2CMasterReadWrite2
  Mux : Mux  Inputs=3
  Mux1 : Mux  Inputs=3
  Old gyro get data Used during SPI before : Subsystem  Commented=on
  Turn the MSB and LSB into a signed 16-bit integer AccX : Subsystem
  Turn the MSB and LSB into a signed 16-bit integer AccY : Subsystem
  Turn the MSB and LSB into a signed 16-bit integer AccZ : Subsystem
  Turn the MSB and LSB into a signed 16-bit integer GyroX : Subsystem
  Turn the MSB and LSB into a signed 16-bit integer GyroY : Subsystem
  Turn the MSB and LSB into a signed 16-bit integer GyroZ : Subsystem
  acc : Outport
  gyro : Outport  Port=2
  wires:
  I2C Master Read/Write2/1 -> DUMMY/1
  Mux/1 -> acc/1
  Turn the MSB and LSB into a signed 16-bit integer AccX/1(out16b) -> Data Type Conversion1/1
  Turn the MSB and LSB into a signed 16-bit integer AccY/1(out16b) -> Data Type Conversion6/1
  Turn the MSB and LSB into a signed 16-bit integer AccZ/1(out16b) -> Data Type Conversion12/1
  Data Type Conversion1/1 -> Mux/1  "ax"
  Data Type Conversion6/1 -> Mux/2  "ay"
  Data Type Conversion12/1 -> Mux/3  "az"
  I2C Master Read/Write1/1 -> DUMMY2/1
  Mux1/1 -> gyro/1
  Turn the MSB and LSB into a signed 16-bit integer GyroX/1(out16b) -> Data Type Conversion16/1
  Turn the MSB and LSB into a signed 16-bit integer GyroY/1(out16b) -> Data Type Conversion18/1
  Turn the MSB and LSB into a signed 16-bit integer GyroZ/1(out16b) -> Data Type Conversion17/1
  Data Type Conversion16/1 -> Mux1/1  "ax"
  Data Type Conversion18/1 -> Mux1/2  "ay"
  Data Type Conversion17/1 -> Mux1/3  "az"
  GYRO_XOUT_H/1 -> I2C Master Read/Write1/2
  ACCEL_XOUT_H/1 -> I2C Master Read/Write2/2
  SlvAddr/1 -> I2C Master Read/Write1/1, I2C Master Read/Write2/1
  I2C Master Read/Write2/2 -> Turn the MSB and LSB into a signed 16-bit integer AccX/1(MSB)  "ACCEL_XOUT_H"
  I2C Master Read/Write2/3 -> Turn the MSB and LSB into a signed 16-bit integer AccX/2(LSB)  "ACCEL_XOUT_L"
  I2C Master Read/Write2/5 -> Turn the MSB and LSB into a signed 16-bit integer AccY/2(LSB)  "ACCEL_YOUT_L"
  I2C Master Read/Write2/4 -> Turn the MSB and LSB into a signed 16-bit integer AccY/1(MSB)  "ACCEL_YOUT_H"
  I2C Master Read/Write2/6 -> Turn the MSB and LSB into a signed 16-bit integer AccZ/1(MSB)  "ACCEL_ZOUT_H"
  I2C Master Read/Write2/7 -> Turn the MSB and LSB into a signed 16-bit integer AccZ/2(LSB)  "ACCEL_ZOUT_L"
  I2C Master Read/Write1/2 -> Turn the MSB and LSB into a signed 16-bit integer GyroX/1(MSB)  "GYRO_XOUT_H"
  I2C Master Read/Write1/3 -> Turn the MSB and LSB into a signed 16-bit integer GyroX/2(LSB)  "GYRO_XOUT_L"
  I2C Master Read/Write1/4 -> Turn the MSB and LSB into a signed 16-bit integer GyroY/1(MSB)  "GYRO_YOUT_H"
  I2C Master Read/Write1/5 -> Turn the MSB and LSB into a signed 16-bit integer GyroY/2(LSB)  "GYRO_YOUT_L"
  I2C Master Read/Write1/6 -> Turn the MSB and LSB into a signed 16-bit integer GyroZ/1(MSB)  "GYRO_ZOUT_H"
  I2C Master Read/Write1/7 -> Turn the MSB and LSB into a signed 16-bit integer GyroZ/2(LSB)  "GYRO_ZOUT_L"

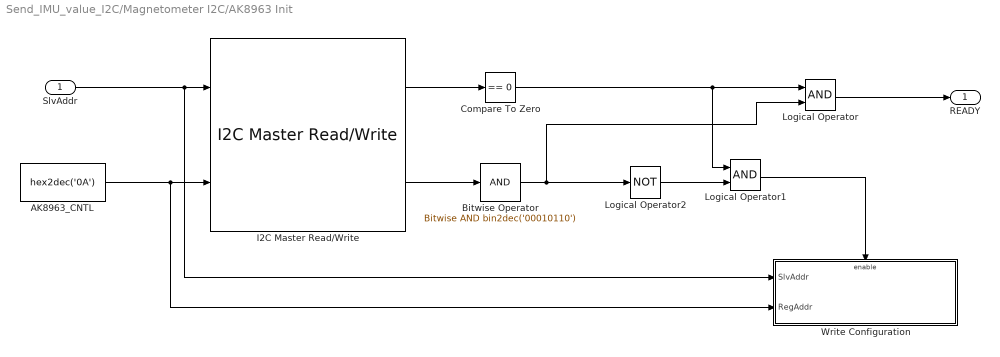
== system Send_IMU_value_I2C/Magnetometer I2C/AK8963 Init  ==
  SlvAddr : Inport
  AK8963_CNTL : Constant  Value=hex2dec('0A')  OutDataTypeStr=uint8  SampleTime=-1
  Bitwise Operator : simulink/Logic and Bit Operations/Bitwise Operator  logicop=AND  UseBitMask=on  BitMask=bin2dec('00010110')  BitMaskRealWorld=Stored Integer
  Compare To Zero : simulink/Logic and Bit Operations/Compare To Zero  relop===  OutDataTypeStr=boolean
  I2C Master Read/Write : stm32f4_i2c_lib/I2C Master Read//Write  configuration=Transaction  module=1  lastmodule=3  transfer=Blocking  dutycycle=TLow/THigh = 2  clkspeed=400  timeout=25  writecount=1  readcount=1  sdapin=C9  sclpin=A8  waitwritetime=0  forcestop=off  inputtypearray=[2 3 3]  outputtypearray=[2 3 3]  confstr="[\"C\",\"9\",\"A\",\"8\",\"1\",\"1\",\"6\",\"0\",\"I2C_DutyCycle_2\",\"0\",\"off\"]"  sampletime=-1  sampletimestr=-1  blockid=MagnetometerI2CAK8963InitI2CMasterReadWrite
  Logical Operator : Logic  AllPortsSameDT=off  OutDataTypeStr=boolean
  Logical Operator1 : Logic  AllPortsSameDT=off  OutDataTypeStr=boolean
  Logical Operator2 : Logic  Operator=NOT  AllPortsSameDT=off  OutDataTypeStr=boolean
  Write Configuration : Subsystem
  READY : Outport
  wires:
  SlvAddr/1 -> Write Configuration/1(SlvAddr), I2C Master Read/Write/1
  AK8963_CNTL/1 -> Write Configuration/2(RegAddr), I2C Master Read/Write/2
  I2C Master Read/Write/1 -> Compare To Zero/1
  Logical Operator/1 -> READY/1
  Bitwise Operator/1 -> Logical Operator2/1, Logical Operator/2
  Compare To Zero/1 -> Logical Operator/1, Logical Operator1/1
  I2C Master Read/Write/2 -> Bitwise Operator/1
  Logical Operator2/1 -> Logical Operator1/2
  Logical Operator1/1 -> Write Configuration/Enable

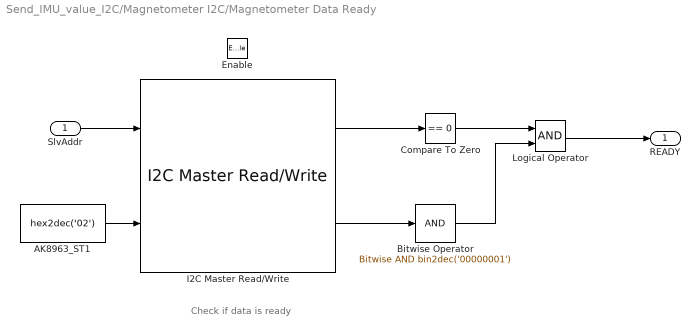
== system Send_IMU_value_I2C/Magnetometer I2C/Magnetometer Data Ready  ==
  note: Check if data is ready
  SlvAddr : Inport
  Enable : EnablePort
  AK8963_ST1 : Constant  Value=hex2dec('02')  OutDataTypeStr=uint8  SampleTime=-1
  Bitwise Operator : simulink/Logic and Bit Operations/Bitwise Operator  logicop=AND  UseBitMask=on  BitMask=bin2dec('00000001')  BitMaskRealWorld=Stored Integer
  Compare To Zero : simulink/Logic and Bit Operations/Compare To Zero  relop===  OutDataTypeStr=boolean
  I2C Master Read/Write : stm32f4_i2c_lib/I2C Master Read//Write  configuration=Transaction  module=1  lastmodule=3  transfer=Blocking  dutycycle=TLow/THigh = 2  clkspeed=400  timeout=25  writecount=1  readcount=1  sdapin=C9  sclpin=A8  waitwritetime=0  forcestop=off  inputtypearray=[2 3 3]  outputtypearray=[2 3 3]  confstr="[\"C\",\"9\",\"A\",\"8\",\"1\",\"1\",\"6\",\"0\",\"I2C_DutyCycle_2\",\"0\",\"off\"]"  sampletime=-1  sampletimestr=-1  blockid=MagnetometerI2CMagnetometerDataReadyI2CMasterReadWrite
  Logical Operator : Logic  AllPortsSameDT=off  OutDataTypeStr=boolean
  READY : Outport
  wires:
  SlvAddr/1 -> I2C Master Read/Write/1
  AK8963_ST1/1 -> I2C Master Read/Write/2
  I2C Master Read/Write/2 -> Bitwise Operator/1
  I2C Master Read/Write/1 -> Compare To Zero/1
  Compare To Zero/1 -> Logical Operator/1
  Bitwise Operator/1 -> Logical Operator/2
  Logical Operator/1 -> READY/1

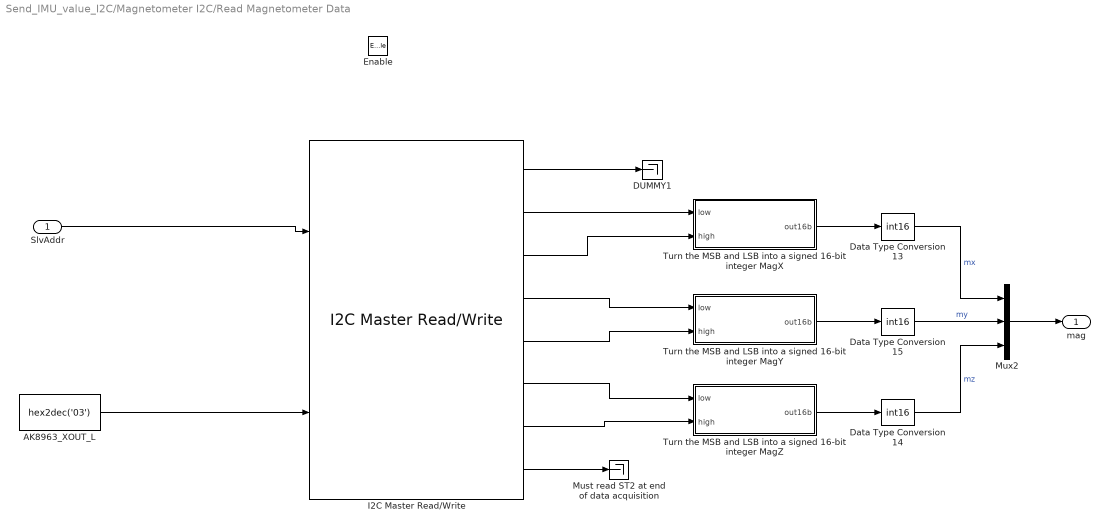
== system Send_IMU_value_I2C/Magnetometer I2C/Read Magnetometer Data ==
  "SlvAddr " : Inport
  Enable : EnablePort
  AK8963_XOUT_L : Constant  Value=hex2dec('03')  OutDataTypeStr=uint8  SampleTime=-1
  DUMMY1 : Terminator
  Data Type Conversion13 : DataTypeConversion  OutDataTypeStr=int16
  Data Type Conversion14 : DataTypeConversion  OutDataTypeStr=int16
  Data Type Conversion15 : DataTypeConversion  OutDataTypeStr=int16
  I2C Master Read/Write : stm32f4_i2c_lib/I2C Master Read//Write  configuration=Transaction  module=1  lastmodule=3  transfer=Blocking  dutycycle=TLow/THigh = 2  clkspeed=400  timeout=25  writecount=1  readcount=7  sdapin=C9  sclpin=A8  waitwritetime=0  forcestop=off  inputtypearray=[2 3 3]  outputtypearray=[8 3 3 3 3 3 3 3 3]  confstr="[\"C\",\"9\",\"A\",\"8\",\"1\",\"1\",\"6\",\"0\",\"I2C_DutyCycle_2\",\"0\",\"off\"]"  sampletime=-1  sampletimestr=-1  blockid=MagnetometerI2CReadMagnetometerDataI2CMasterReadWrite
  "Must read ST2 at end of data acquisition  " : Terminator
  Mux2 : Mux  Inputs=3
  Turn the MSB and LSB into a signed 16-bit integer MagX : Subsystem
  Turn the MSB and LSB into a signed 16-bit integer MagY : Subsystem
  Turn the MSB and LSB into a signed 16-bit integer MagZ : Subsystem
  mag : Outport
  wires:
  Turn the MSB and LSB into a signed 16-bit integer MagX/1(out16b) -> Data Type Conversion13/1
  Turn the MSB and LSB into a signed 16-bit integer MagY/1(out16b) -> Data Type Conversion15/1
  Turn the MSB and LSB into a signed 16-bit integer MagZ/1(out16b) -> Data Type Conversion14/1
  Data Type Conversion13/1 -> Mux2/1  "mx"
  Data Type Conversion15/1 -> Mux2/2  "my"
  Data Type Conversion14/1 -> Mux2/3  "mz"
  AK8963_XOUT_L/1 -> I2C Master Read/Write/2
  I2C Master Read/Write/1 -> DUMMY1/1
  "SlvAddr "/1 -> I2C Master Read/Write/1
  Mux2/1 -> mag/1
  I2C Master Read/Write/8 -> "Must read ST2 at end of data acquisition  "/1
  I2C Master Read/Write/3 -> Turn the MSB and LSB into a signed 16-bit integer MagX/2(high)
  I2C Master Read/Write/2 -> Turn the MSB and LSB into a signed 16-bit integer MagX/1(low)
  I2C Master Read/Write/4 -> Turn the MSB and LSB into a signed 16-bit integer MagY/1(low)
  I2C Master Read/Write/5 -> Turn the MSB and LSB into a signed 16-bit integer MagY/2(high)
  I2C Master Read/Write/6 -> Turn the MSB and LSB into a signed 16-bit integer MagZ/1(low)
  I2C Master Read/Write/7 -> Turn the MSB and LSB into a signed 16-bit integer MagZ/2(high)

== system Send_IMU_value_I2C/Accelometer Gyroscope I2C/MPU9250 Init/Write Configuration ==
  SlvAddr : Inport
  Enable : EnablePort
  BYPASS_EN : Constant  Value=hex2dec('02')  OutDataTypeStr=uint8  SampleTime=-1
  I2C Master Read/Write1 : stm32f4_i2c_lib/I2C Master Read//Write  configuration=Transaction  module=1  lastmodule=3  transfer=Blocking  dutycycle=TLow/THigh = 2  clkspeed=400  timeout=25  writecount=2  readcount=0  sdapin=C9  sclpin=A8  waitwritetime=0  forcestop=off  inputtypearray=[3 3 3 3]  outputtypearray=[1 3]  confstr="[\"C\",\"9\",\"A\",\"8\",\"1\",\"1\",\"6\",\"0\",\"I2C_DutyCycle_2\",\"0\",\"off\"]"  sampletime=-1  sampletimestr=-1  blockid=AccelometerGyroscopeI2CMPU9250InitWriteConfigurationI2CMasterReadWrite1
  INT_PIN_CFG1 : Constant  Value=hex2dec('37')  OutDataTypeStr=uint8  SampleTime=-1
  Terminator : Terminator
  wires:
  I2C Master Read/Write1/1 -> Terminator/1
  BYPASS_EN/1 -> I2C Master Read/Write1/3
  INT_PIN_CFG1/1 -> I2C Master Read/Write1/2
  SlvAddr/1 -> I2C Master Read/Write1/1
